simulink model "adaptiveIPDComboCtrl"  (R2016b)
settings: Solver=ode5  StartTime=0.0  StopTime=12*pi  FixedStep=0.001  RelTol=1e-3  EnableMultiTasking=on
undefined symbols (not defined in the file or in its folder): Humusoft, MF644
libraries: dcpctrl x2, simulink x1, sldrtlib x1
settings Model: SimulationMode=external  Creator=julianleland  LastModifiedBy=julianleland
settings OptimizationCC: LifeSpan=inf
settings DebuggingCC: SFUnexpectedBacktrackingDiag=warning  SFNoUnconditionalDefaultTransitionDiag=warning  SFExecutionAtInitializationDiag=none
settings HardwareCC: ProdBitPerLong=64  ProdHWDeviceType=Intel->x86-64 (Mac OS X)  TargetBitPerLong=64  TargetBitPerPointer=64  TargetIntDivRoundTo=Zero  TargetEndianess=LittleEndian  TargetWordSize=64  TargetHWDeviceType=Intel->x86-64
settings RTWCC: SystemTargetFile=sldrt.tlc  TemplateMakefile=sldrt.tmf  Description=Simulink Desktop Real-Time  RTWCompilerOptimization=on
settings CodeAppCC: MaxIdLength=95
settings SimulinkDesktopRealTimeCC: TargetPreCompLibLocation=/Applications/MATLAB_R2016b.app/toolbox/sldrt/lib/maci64  TargetLangStandard=C89/C90 (ANSI)  SupportVariableSizeSignals=off
settings ConfigComp: CovMetricSettings=dw  CovHtmlReporting=on  CovSaveCumulativeToWorkspaceVar=on  CovSaveSingleToWorkspaceVar=on  CovExternalEMLEnable=off

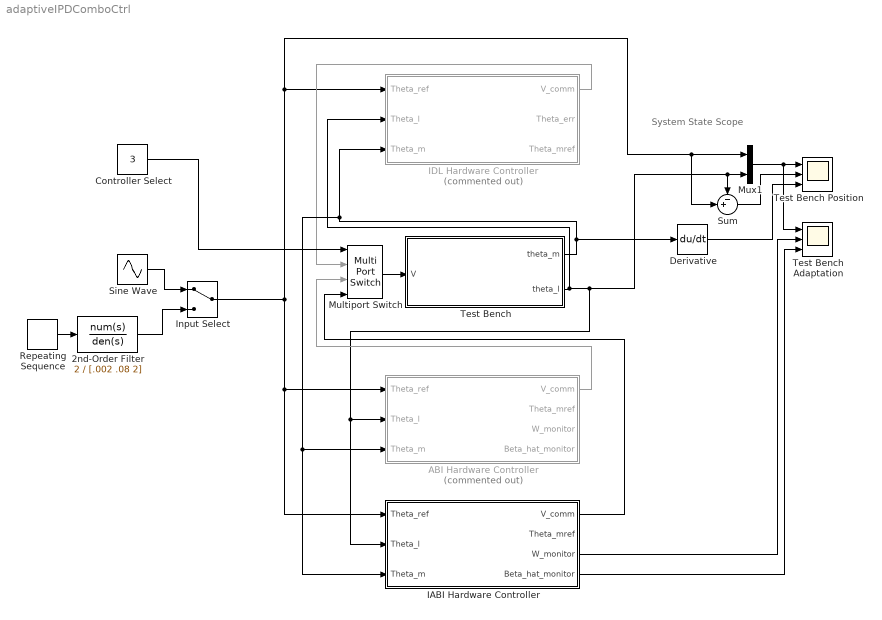
== system adaptiveIPDComboCtrl ==
  note: System State Scope
  2nd-Order Filter : TransferFcn  Numerator=2  Denominator=[.002 .08 2]
  ABI Hardware Controller : Subsystem  Commented=on
  Controller Select : Constant  Value=3
  Derivative : Derivative
  IABI Hardware Controller : Subsystem
  IDL Hardware Controller : Subsystem  Commented=on
  Input Select : ManualSwitch
  Multiport Switch : MultiPortSwitch
  Mux1 : Mux  Inputs=2
  Repeating Sequence : simulink/Sources/Repeating Sequence  rep_seq_t=3*[0 1 1.05 1.1 2 2.05 2.1]  rep_seq_y=[0 0 1 2 2 1 0 ]
  Sine Wave : Sin  Amplitude=2  SampleTime=0
  Sum : Sum  Inputs=-+|
  Test Bench : Subsystem
  Test Bench Adaptation : Scope  NumInputPorts=3
  Test Bench Position : Scope  NumInputPorts=3
  wires:
  Mux1/1 -> Test Bench Adaptation/1, Test Bench Position/1
  Sum/1 -> Test Bench Position/2
  Input Select/1 -> IDL Hardware Controller/1(Theta_ref), Sum/2, Mux1/1, IABI Hardware Controller/1(Theta_ref), ABI Hardware Controller/1(Theta_ref)
  Sine Wave/1 -> Input Select/1
  IABI Hardware Controller/4(Beta_hat_monitor) -> Test Bench Adaptation/3
  IABI Hardware Controller/3(W_monitor) -> Test Bench Adaptation/2
  IDL Hardware Controller/1(V_comm) -> Multiport Switch/2
  Test Bench/2(theta_l) -> IABI Hardware Controller/2(Theta_l), ABI Hardware Controller/2(Theta_l), Sum/1, Mux1/2, IDL Hardware Controller/2(Theta_l)
  Multiport Switch/1 -> Test Bench/1(V)
  Test Bench/1(theta_m) -> Derivative/1, IABI Hardware Controller/3(Theta_m), ABI Hardware Controller/3(Theta_m), IDL Hardware Controller/3(Theta_m)
  Derivative/1 -> Test Bench Position/3
  ABI Hardware Controller/1(V_comm) -> Multiport Switch/3
  IABI Hardware Controller/1(V_comm) -> Multiport Switch/4
  Controller Select/1 -> Multiport Switch/1
  Repeating Sequence/1 -> 2nd-Order Filter/1
  2nd-Order Filter/1 -> Input Select/2

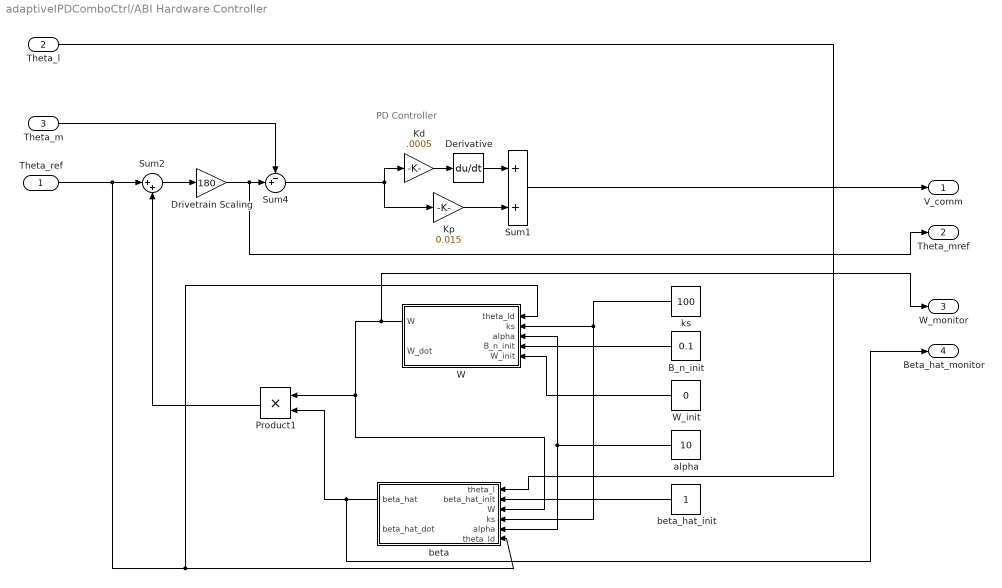
== system adaptiveIPDComboCtrl/ABI Hardware Controller ==
  note: PD Controller
  Theta_ref : Inport
  Theta_l : Inport  Port=2
  Theta_m : Inport  Port=3
  B_n_init : Constant  Value=0.1
  Derivative : Derivative
  Drivetrain Scaling : Gain  Gain=180
  Kd : Gain  Gain=.0005
  Kp : Gain  Gain=0.015
  Product1 : Product
  Sum1 : Sum
  Sum2 : Sum  Inputs=|++
  Sum4 : Sum  Inputs=-+|
  W : Subsystem
  W_init : Constant  Value=0
  alpha : Constant  Value=10
  beta : Subsystem
  beta_hat_init : Constant
  ks : Constant  Value=100
  V_comm : Outport
  Theta_mref : Outport  Port=2
  W_monitor : Outport  Port=3
  Beta_hat_monitor : Outport  Port=4
  wires:
  Sum2/1 -> Drivetrain Scaling/1
  Theta_ref/1 -> W/1(theta_ld), beta/6(theta_ld), Sum2/1
  beta_hat_init/1 -> beta/2(beta_hat_init)
  beta/1(beta_hat) -> Beta_hat_monitor/1, Product1/2
  alpha/1 -> beta/5(alpha), W/3(alpha)
  Kp/1 -> Sum1/2
  Kd/1 -> Derivative/1
  ks/1 -> beta/4(ks), W/2(ks)
  W/1(W) -> W_monitor/1, beta/3(W), Product1/1
  B_n_init/1 -> W/4(B_n_init)
  W_init/1 -> W/5(W_init)
  Sum4/1 -> Kp/1, Kd/1
  Derivative/1 -> Sum1/1
  Drivetrain Scaling/1 -> Theta_mref/1, Sum4/2
  Product1/1 -> Sum2/2
  Theta_l/1 -> beta/1(theta_l)
  Sum1/1 -> V_comm/1
  Theta_m/1 -> Sum4/1

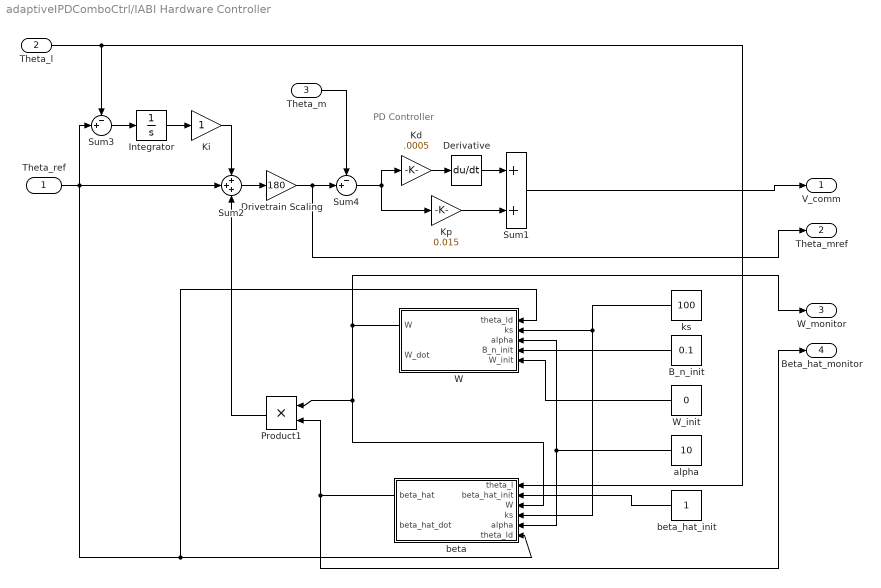
== system adaptiveIPDComboCtrl/IABI Hardware Controller ==
  note: PD Controller
  Theta_ref : Inport
  Theta_l : Inport  Port=2
  Theta_m : Inport  Port=3
  B_n_init : Constant  Value=0.1
  Derivative : Derivative
  Drivetrain Scaling : Gain  Gain=180
  Integrator : Integrator  LimitOutput=on  UpperSaturationLimit=10  LowerSaturationLimit=-10
  Kd : Gain  Gain=.0005
  Ki : Gain
  Kp : Gain  Gain=0.015
  Product1 : Product  Inputs=**
  Sum1 : Sum
  Sum2 : Sum  Inputs=+++
  Sum3 : Sum  Inputs=-+|
  Sum4 : Sum  Inputs=-+|
  W : Subsystem
  W_init : Constant  Value=0
  alpha : Constant  Value=10
  beta : Subsystem
  beta_hat_init : Constant
  ks : Constant  Value=100
  V_comm : Outport
  Theta_mref : Outport  Port=2
  W_monitor : Outport  Port=3
  Beta_hat_monitor : Outport  Port=4
  wires:
  Theta_m/1 -> Sum4/1
  Sum1/1 -> V_comm/1
  Theta_l/1 -> beta/1(theta_l), Sum3/1
  Product1/1 -> Sum2/3
  Drivetrain Scaling/1 -> Sum4/2, Theta_mref/1
  Derivative/1 -> Sum1/1
  Sum4/1 -> Kd/1, Kp/1
  W_init/1 -> W/5(W_init)
  B_n_init/1 -> W/4(B_n_init)
  W/1(W) -> Product1/1, beta/3(W), W_monitor/1
  ks/1 -> W/2(ks), beta/4(ks)
  Kd/1 -> Derivative/1
  Kp/1 -> Sum1/2
  alpha/1 -> W/3(alpha), beta/5(alpha)
  beta/1(beta_hat) -> Beta_hat_monitor/1, Product1/2
  beta_hat_init/1 -> beta/2(beta_hat_init)
  Theta_ref/1 -> Sum3/2, Sum2/2, beta/6(theta_ld), W/1(theta_ld)
  Sum2/1 -> Drivetrain Scaling/1
  Sum3/1 -> Integrator/1
  Integrator/1 -> Ki/1
  Ki/1 -> Sum2/1

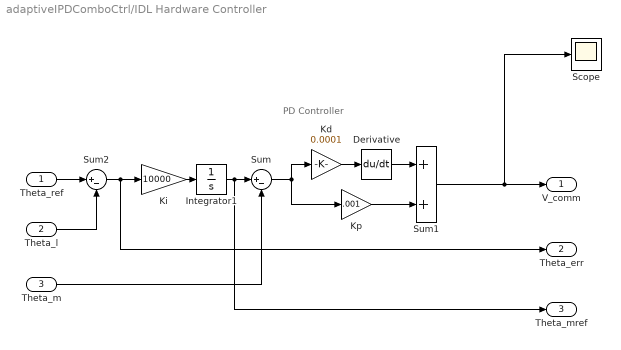
== system adaptiveIPDComboCtrl/IDL Hardware Controller ==
  note: PD Controller
  Theta_ref : Inport
  Theta_l : Inport  Port=2
  Theta_m : Inport  Port=3
  Derivative : Derivative
  Integrator1 : Integrator  LimitOutput=on  UpperSaturationLimit=2000  LowerSaturationLimit=-2000
  Kd : Gain  Gain=0.0001
  Ki : Gain  Gain=10000
  Kp : Gain  Gain=.001
  Scope : Scope
  Sum : Sum  Inputs=|+-
  Sum1 : Sum
  Sum2 : Sum  Inputs=|+-
  V_comm : Outport
  Theta_err : Outport  Port=2
  Theta_mref : Outport  Port=3
  wires:
  Integrator1/1 -> Theta_mref/1, Sum/1
  Theta_ref/1 -> Sum2/1
  Kd/1 -> Derivative/1
  Sum/1 -> Kp/1, Kd/1
  Derivative/1 -> Sum1/1
  Kp/1 -> Sum1/2
  Ki/1 -> Integrator1/1
  Sum2/1 -> Theta_err/1, Ki/1
  Sum1/1 -> V_comm/1, Scope/1
  Theta_l/1 -> Sum2/2
  Theta_m/1 -> Sum/2

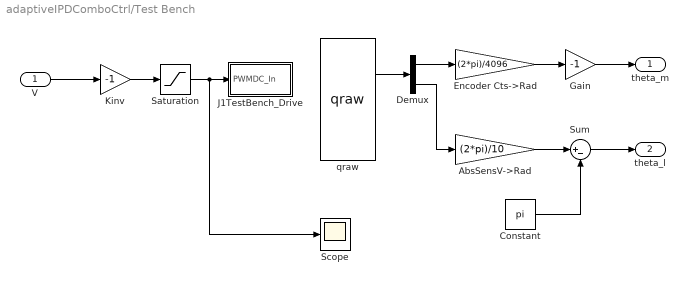
== system adaptiveIPDComboCtrl/Test Bench ==
  V : Inport
  AbsSensV->Rad : Gain  Gain=(2*pi)/10
  Constant : Constant  Value=pi
  Demux : Demux  Outputs=2
  Encoder Cts->Rad : Gain  Gain=(2*pi)/4096
  Gain : Gain  Gain=-1
  J1TestBench_Drive : Subsystem
  Kinv : Gain  Gain=-1
  Saturation : Saturate  UpperLimit=1  LowerLimit=-1
  Scope : Scope
  Sum : Sum  Inputs=|+-
  qraw : dcpctrl/qraw
  theta_m : Outport
  theta_l : Outport  Port=2
  wires:
  Gain/1 -> theta_m/1
  Encoder Cts->Rad/1 -> Gain/1
  Constant/1 -> Sum/2
  Sum/1 -> theta_l/1
  AbsSensV->Rad/1 -> Sum/1
  qraw/2 -> Demux/1
  V/1 -> Kinv/1
  Demux/2 -> AbsSensV->Rad/1
  Kinv/1 -> Saturation/1
  Demux/1 -> Encoder Cts->Rad/1
  Saturation/1 -> J1TestBench_Drive/1(PWMDC_In), Scope/1

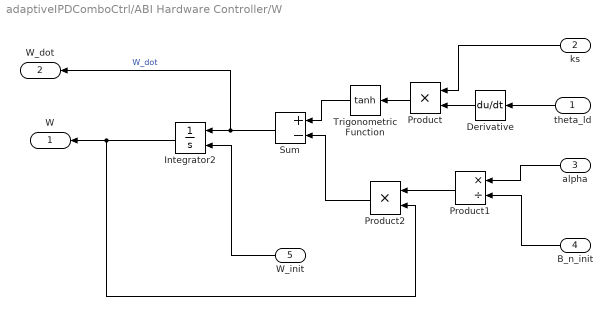
== system adaptiveIPDComboCtrl/ABI Hardware Controller/W ==
  theta_ld : Inport
  ks : Inport  Port=2
  alpha : Inport  Port=3
  B_n_init : Inport  Port=4
  W_init : Inport  Port=5
  Derivative : Derivative
  Integrator2 : Integrator  InitialConditionSource=external
  Product : Product
  Product1 : Product  Inputs=*/
  Product2 : Product
  Sum : Sum  Inputs=+-
  Trigonometric Function : Trigonometry  Operator=tanh
  W : Outport
  W_dot : Outport  Port=2
  wires:
  Product2/1 -> Sum/2
  W_init/1 -> Integrator2/2
  Sum/1 -> Integrator2/1, W_dot/1  "W_dot"
  Trigonometric Function/1 -> Sum/1
  theta_ld/1 -> Derivative/1
  Product/1 -> Trigonometric Function/1
  Product1/1 -> Product2/1
  B_n_init/1 -> Product1/2
  alpha/1 -> Product1/1
  ks/1 -> Product/1
  Derivative/1 -> Product/2
  Integrator2/1 -> W/1, Product2/2

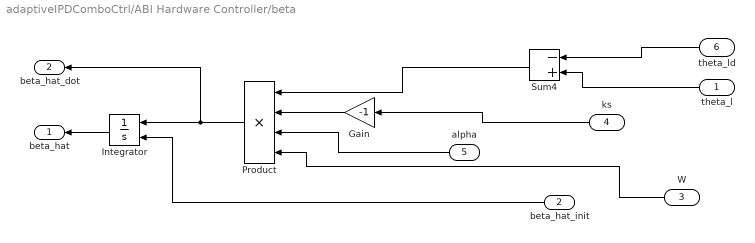
== system adaptiveIPDComboCtrl/ABI Hardware Controller/beta ==
  theta_l : Inport
  beta_hat_init : Inport  Port=2
  W : Inport  Port=3
  ks : Inport  Port=4
  alpha : Inport  Port=5
  theta_ld : Inport  Port=6
  Gain : Gain  Gain=-1
  Integrator : Integrator  InitialConditionSource=external
  Product : Product  Inputs=****
  Sum4 : Sum  Inputs=-+
  beta_hat : Outport
  beta_hat_dot : Outport  Port=2
  wires:
  beta_hat_init/1 -> Integrator/2
  Integrator/1 -> beta_hat/1
  ks/1 -> Gain/1
  theta_ld/1 -> Sum4/1
  theta_l/1 -> Sum4/2
  alpha/1 -> Product/3
  W/1 -> Product/4
  Gain/1 -> Product/2
  Product/1 -> beta_hat_dot/1, Integrator/1
  Sum4/1 -> Product/1

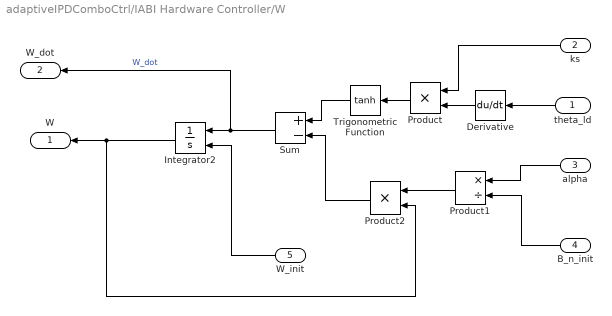
== system adaptiveIPDComboCtrl/IABI Hardware Controller/W ==
  theta_ld : Inport
  ks : Inport  Port=2
  alpha : Inport  Port=3
  B_n_init : Inport  Port=4
  W_init : Inport  Port=5
  Derivative : Derivative
  Integrator2 : Integrator  InitialConditionSource=external
  Product : Product
  Product1 : Product  Inputs=*/
  Product2 : Product
  Sum : Sum  Inputs=+-
  Trigonometric Function : Trigonometry  Operator=tanh
  W : Outport
  W_dot : Outport  Port=2
  wires:
  Integrator2/1 -> Product2/2, W/1
  Derivative/1 -> Product/2
  ks/1 -> Product/1
  alpha/1 -> Product1/1
  B_n_init/1 -> Product1/2
  Product1/1 -> Product2/1
  Product/1 -> Trigonometric Function/1
  theta_ld/1 -> Derivative/1
  Trigonometric Function/1 -> Sum/1
  Sum/1 -> W_dot/1, Integrator2/1  "W_dot"
  W_init/1 -> Integrator2/2
  Product2/1 -> Sum/2

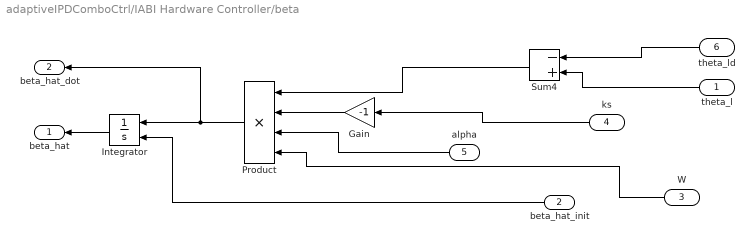
== system adaptiveIPDComboCtrl/IABI Hardware Controller/beta ==
  theta_l : Inport
  beta_hat_init : Inport  Port=2
  W : Inport  Port=3
  ks : Inport  Port=4
  alpha : Inport  Port=5
  theta_ld : Inport  Port=6
  Gain : Gain  Gain=-1
  Integrator : Integrator  InitialConditionSource=external
  Product : Product  Inputs=****
  Sum4 : Sum  Inputs=-+
  beta_hat : Outport
  beta_hat_dot : Outport  Port=2
  wires:
  Product/1 -> Integrator/1, beta_hat_dot/1
  Gain/1 -> Product/2
  W/1 -> Product/4
  alpha/1 -> Product/3
  theta_l/1 -> Sum4/2
  theta_ld/1 -> Sum4/1
  ks/1 -> Gain/1
  Integrator/1 -> beta_hat/1
  beta_hat_init/1 -> Integrator/2
  Sum4/1 -> Product/1

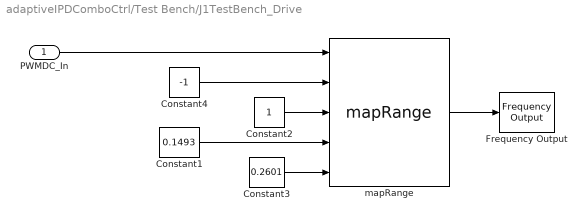
== system adaptiveIPDComboCtrl/Test Bench/J1TestBench_Drive ==
  PWMDC_In : Inport
  Constant1 : Constant  Value=0.1493
  Constant2 : Constant
  Constant3 : Constant  Value=0.2601
  Constant4 : Constant  Value=-1
  Frequency Output : sldrtlib/Frequency Output  SampleTime=-1  MaxMissedTicks=10  ShowMissedTicks=off  YieldWhenWaiting=off  DrvName=Humusoft/MF644  DrvAddress=4294967295  DrvOptions=585  Channels=1  FrequencySource=1  Frequency=150  FrequencyFinalValue=[]  DutySource=2  Duty=0.5  DutyFinalValue=0.5
      settings: AttributesFormatString=Humusoft\nMF644 [auto]
  "mapRange " : dcpctrl/mapRange 
  wires:
  Constant2/1 -> "mapRange "/3
  Constant3/1 -> "mapRange "/5
  Constant4/1 -> "mapRange "/2
  PWMDC_In/1 -> "mapRange "/1
  "mapRange "/1 -> Frequency Output/1
  Constant1/1 -> "mapRange "/4
